simulink model "KiemTraDongHoc"  (R2022b)
settings: Solver=VariableStepAuto  StartTime=0.0  StopTime=10.0  RelTol=1e-3
settings Model: Creator=at632  LastModifiedBy=at632

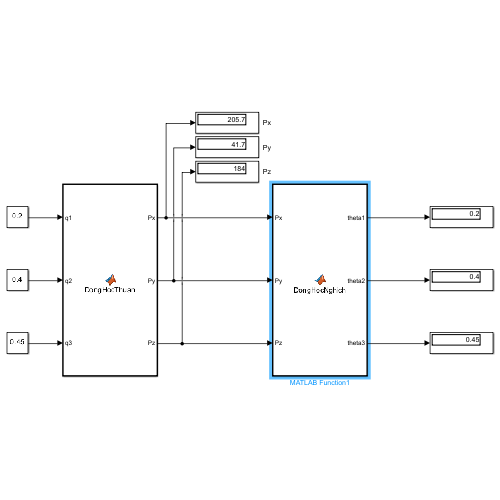
[thumbnail: Simulink's stored preview of the top-level diagram]
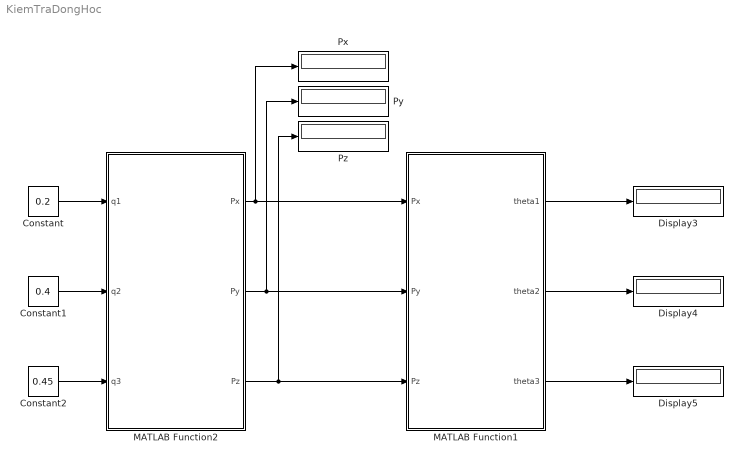
== system KiemTraDongHoc ==
  Constant : Constant  Value=0.2
  Constant1 : Constant  Value=0.4
  Constant2 : Constant  Value=0.45
  Display3 : Display
  Display4 : Display
  Display5 : Display
  MATLAB Function1 : MATLAB Function  TreatAsAtomicUnit=on
  MATLAB Function2 : MATLAB Function  TreatAsAtomicUnit=on
  Px : Display
  Py : Display
  Pz : Display
  wires:
  MATLAB Function2/1(Px) -> MATLAB Function1/1(Px), Px/1
  MATLAB Function2/2(Py) -> MATLAB Function1/2(Py), Py/1
  MATLAB Function2/3(Pz) -> MATLAB Function1/3(Pz), Pz/1
  MATLAB Function1/1(theta1) -> Display3/1
  MATLAB Function1/2(theta2) -> Display4/1
  MATLAB Function1/3(theta3) -> Display5/1
  Constant/1 -> MATLAB Function2/1(q1)
  Constant1/1 -> MATLAB Function2/2(q2)
  Constant2/1 -> MATLAB Function2/3(q3)

== matlab function KiemTraDongHoc/MATLAB Function1 ==
  data: Px input; theta1 output; Py input; Pz input; theta2 output; theta3 output
function [theta1, theta2, theta3] = DongHocNghich(Px,Py,Pz)

l1=150;
l2=200;
l3=200;

theta1 = atan2(Py, Px);
theta2 =  -2*atan((((- Px^2 - Py^2 - Pz^2 + 2*Pz*l1 - l1^2 + l2^2 + 2*l2*l3 + l3^2)* ...
    (Px^2 + Py^2 + Pz^2 - 2*Pz*l1 + l1^2 - l2^2 + 2*l2*l3 - l3^2))^(1/2) - 2*l2*(Px^2 + Py^2)^(1/2))/ ...
    (Px^2 + Py^2 + Pz^2 - 2*Pz*l1 + 2*Pz*l2 + l1^2 - 2*l1*l2 + l2^2 - l3^2));
theta3 =  -2*atan((2*l2*l3 - ((- Px^2 - Py^2 - Pz^2 + 2*Pz*l1 - l1^2 + l2^2 + 2*l2*l3 + l3^2)* ...
    (Px^2 + Py^2 + Pz^2 - 2*Pz*l1 + l1^2 - l2^2 + 2*l2*l3 - l3^2))^(1/2))/ ...
    (Px^2 + Py^2 + Pz^2 - 2*Pz*l1 + l1^2 - l2^2 - l3^2));

== matlab function KiemTraDongHoc/MATLAB Function2 ==
  data: q1 input; Px output; q2 input; q3 input; Py output; Pz output
function [Px, Py, Pz] = DongHocThuan(q1,q2,q3)
l1=150;
l2=200;
l3=200;
Px = cos(q1)*(l3*cos(q2 + q3) + l2*sin(q2));
Py = sin(q1)*(l3*cos(q2 + q3) + l2*sin(q2));
Pz =   l1 - l3*sin(q2 + q3) + l2*cos(q2);
